simulink model "cordic_mix_v2"  (R2021a)
settings: Solver=VariableStepAuto  StartTime=0.0  StopTime=500  RelTol=1e-3
libraries: xbsIndex_r4 x68, dspsrcs4 x6
settings Model: Creator=user  LastModifiedBy=11037
settings SolverCC: AlgebraicLoopSolver=TrustRegion
settings DataIOCC: ReturnWorkspaceOutputs=off
settings DebuggingCC: SFMachineParentedDataDiag=warning

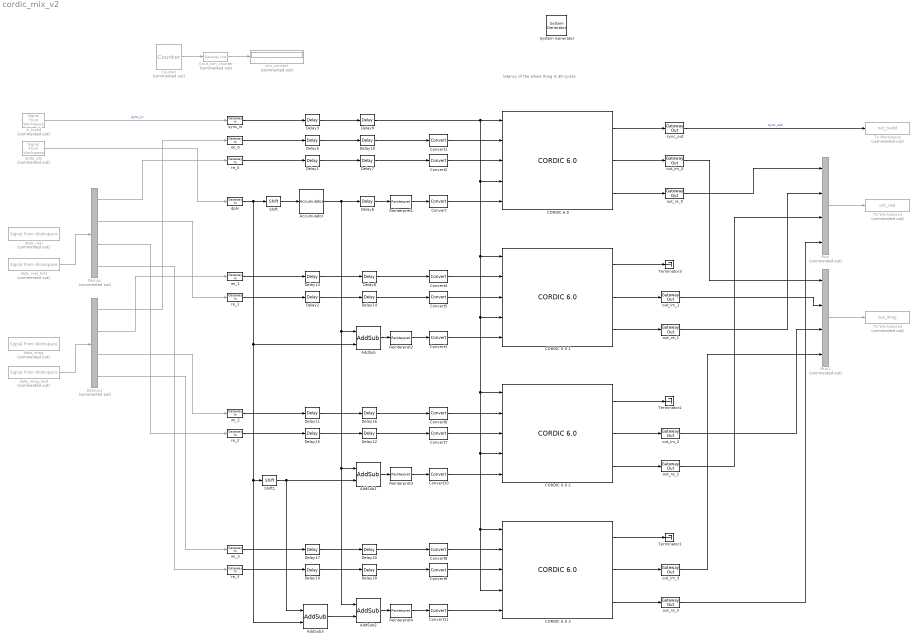
== system cordic_mix_v2 ==
  note: latency of the whole thing is 30 cycles
  " System Generator" : xbsIndex_r4/ System Generator  Tag=genX  xilinxfamily=zynquplusRFSOC  part=xczu28dr  speed=-2-e  package=ffvg1517  synthesis_tool=Vivado  clock_wrapper=Clock Enables  directory=C:/cordic_mix_v2_NL  proj_type=Vivado  Synth_file=Vivado Synthesis Defaults  Impl_file=Vivado Implementation Defaults  testbench=off  simulink_period=1  sysclk_period=10  dcm_input_clock_period=10  incr_netlist=off  trim_vbits=Everywhere in SubSystem  dbl_ovrd=According to Block Masks  core_generation=According to Block Masks  run_coregen=off  deprecated_control=off  eval_field=0  block_type=sysgen
  Accumulator : xbsIndex_r4/Accumulator  operation=Add  n_bits=22  overflow=Wrap  scale=1  rst=off  hasbypass=off  infoeditControl=reset for floating point data type must be asserted for a minimum of 2 cycles  en=off  latency=1  msb_inp=100  msb=100  lsb=-100  use_behavioral_HDL=on  implementation=Fabric  dbl_ovrd=off  block_type=accum
  AddSub : xbsIndex_r4/AddSub  mode=Addition  use_carryin=off  use_carryout=off  en=off  latency=2  precision=User Defined  arith_type=Unsigned  n_bits=22  bin_pt=0  quantization=Truncate  overflow=Wrap  use_behavioral_HDL=off  hw_selection=Fabric  pipelined=off  dbl_ovrd=off  block_type=addsub
  AddSub1 : xbsIndex_r4/AddSub  mode=Addition  use_carryin=off  use_carryout=off  en=off  latency=2  precision=User Defined  arith_type=Unsigned  n_bits=22  bin_pt=0  quantization=Truncate  overflow=Wrap  use_behavioral_HDL=off  hw_selection=Fabric  pipelined=off  dbl_ovrd=off  block_type=addsub
  AddSub2 : xbsIndex_r4/AddSub  mode=Addition  use_carryin=off  use_carryout=off  en=off  latency=2  precision=User Defined  arith_type=Unsigned  n_bits=22  bin_pt=0  quantization=Truncate  overflow=Wrap  use_behavioral_HDL=off  hw_selection=Fabric  pipelined=off  dbl_ovrd=off  block_type=addsub
  AddSub3 : xbsIndex_r4/AddSub  mode=Addition  use_carryin=off  use_carryout=off  en=off  latency=1  precision=User Defined  arith_type=Unsigned  n_bits=22  bin_pt=0  quantization=Truncate  overflow=Wrap  use_behavioral_HDL=off  hw_selection=Fabric  pipelined=off  dbl_ovrd=off  block_type=addsub
  CORDIC 6.0 {,1..3} (4 alike) : xbsIndex_r4/CORDIC 6.0   functional_selection=Rotate  architectural_configuration=Parallel  pipelining_mode=Maximum  data_format=SignedFraction  phase_format=Scaled_Radians  input_width=24  output_width=16  round_mode=Truncate  iterations=18  precision=20  compensation_scaling=LUT_based  coarse_rotation=on  aclken=off  aresetn=off  out_tready=off  cartesian_has_tuser=off  cartesian_has_tlast=off  cartesian_tuser_width=1  phase_has_tuser=off  phase_has_tlast=off  phase_tuser_width=1  out_tlast_behv=Null  flow_control=NonBlocking  optimize_goal=Resources  trim_axipin_name=on  simulation_type=hybrid_sim  simulation_model=sysgen:cordic_v6_0  data_path_portlist={'s_axis_cartesian_tdata_imag', 's_axis_cartesian_tdata_real', 's_axis_phase_tdata_phase', 'm_axis_dout_tdata_imag', 'm_axis_dout_tdata_real', 'm_axis_dout_tdata_phase','m_axis_dout_tdata'}  ip_name=CORDIC  ip_version=6.0  dsptool_ready=true  ipcore_usecache=true  ipcore_useipmodelcache=true  wrapper_available=true  port_translation_map={ 'aclken' => 'en', 'aresetn' => 'rst' }  block_type=cordic_v6_0
      settings: infoedit=CORDIC 6.0
  Convert{,3,10..11} (4 alike) : xbsIndex_r4/Convert  gui_display_data_type=Fixed-point  arith_type="Signed  (2's comp)"  n_bits=24  bin_pt=21  float_type=Single  exp_bits=8  fraction_bits=24  quantization=Truncate  overflow=Flag as error  en=off  latency=0  pipeline=off  dbl_ovrd=off  block_type=convert
  Convert{1..2,4..9} (8 alike) : xbsIndex_r4/Convert  gui_display_data_type=Fixed-point  arith_type="Signed  (2's comp)"  n_bits=24  bin_pt=22  float_type=Single  exp_bits=8  fraction_bits=24  quantization=Truncate  overflow=Flag as error  en=off  latency=0  pipeline=off  dbl_ovrd=off  block_type=convert
  Counter : xbsIndex_r4/Counter  Commented=on  cnt_type=Free Running  cnt_to=Inf  operation=Up  start_count=0  cnt_by_val=1  arith_type=Unsigned  n_bits=24  bin_pt=0  load_pin=off  rst=off  en=off  explicit_period=on  period=1  use_behavioral_HDL=off  implementation=Fabric  dbl_ovrd=off  block_type=counter
  Delay{1..3,5,11,13,15,17,19} (9 alike) : xbsIndex_r4/Delay  rst=off  infoeditControl=Selection of Reset will increase slice count due to use of real FFs and instead of SRLs  en=off  latency=1  reg_retiming=off  dbl_ovrd=off  block_type=delay
  Delay{6..10,12,14,16,18,20} (10 alike) : xbsIndex_r4/Delay  rst=off  infoeditControl=Selection of Reset will increase slice count due to use of real FFs and instead of SRLs  en=off  latency=2  reg_retiming=off  dbl_ovrd=off  block_type=delay
  Demux : Demux  Commented=on
  Demux1 : Demux  Commented=on
  Gout_sim_counter : xbsIndex_r4/Gateway Out  Commented=on  inherit_from_input=on  hdl_port=on  rows=1  columns=1  UseAsDAC=off  DACChannel='1'  interface=None  automatic_assignment=on  address_offset=hex2dec('00')  intf_name=''  intf_description=''  timing_constraint=None  locs_specified=off  LOCs={}  io_standard={}  block_type=gatewayout
  Mux : Mux  Commented=on
  Mux1 : Mux  Commented=on
  Reinterpret{1..4} (4 alike) : xbsIndex_r4/Reinterpret  force_arith_type=on  arith_type="Signed  (2's comp)"  force_bin_pt=on  bin_pt=21  block_type=reinterpret
  Shift : xbsIndex_r4/Shift  shift_dir=Left  shift_bits=2  en=off  latency=0  precision=Full  arith_type="Signed  (2's comp)"  n_bits=16  bin_pt=14  quantization=Truncate  overflow=Wrap  dbl_ovrd=off  block_type=shift
  Shift1 : xbsIndex_r4/Shift  shift_dir=Left  shift_bits=1  en=off  latency=0  precision=Full  arith_type="Signed  (2's comp)"  n_bits=16  bin_pt=14  quantization=Truncate  overflow=Wrap  dbl_ovrd=off  block_type=shift
  Terminator1 : Terminator
  Terminator2 : Terminator
  Terminator3 : Terminator
  To Workspace : ToWorkspace  Commented=on  VariableName=out_tvalid  SampleTime=1
  To Workspace1 : ToWorkspace  Commented=on  VariableName=out_real  SampleTime=1
  To Workspace2 : ToWorkspace  Commented=on  VariableName=out_imag  SampleTime=1
  data_imag : dspsrcs4/Signal From Workspace  Commented=on  X=PSB_out_im_trimmed  Ts=1  nsamps=1  OutputAfterFinalValue=Cyclic repetition  ignoreOrWarnInputAndFrameLengths=off  OutputFrames=off
  data_imag_test : dspsrcs4/Signal From Workspace  Commented=on  X=cordic_test_signal_imag  Ts=1  nsamps=1  OutputAfterFinalValue=Cyclic repetition  ignoreOrWarnInputAndFrameLengths=off  OutputFrames=off
  data_real : dspsrcs4/Signal From Workspace  Commented=on  X=PSB_out_re_trimmed  Ts=1  nsamps=1  OutputAfterFinalValue=Cyclic repetition  ignoreOrWarnInputAndFrameLengths=off  OutputFrames=off
  data_real_test : dspsrcs4/Signal From Workspace  Commented=on  X=cordic_test_signal_real  Ts=1  nsamps=1  OutputAfterFinalValue=Cyclic repetition  ignoreOrWarnInputAndFrameLengths=off  OutputFrames=off
  delta_phi : dspsrcs4/Signal From Workspace  Commented=on  X=dphi  Ts=1  nsamps=1  OutputAfterFinalValue=Holding final value  ignoreOrWarnInputAndFrameLengths=off  OutputFrames=off
  dphi : xbsIndex_r4/Gateway In  gui_display_data_type=Fixed-point  arith_type=Unsigned  n_bits=22  bin_pt=0  preci_type=Single  exp_width=8  frac_width=24  rows=1  columns=1  quantization=Truncate  overflow=Flag as error  period=1  UseAsADC=off  ADCChannel='1'  interface=None  automatic_assignment=on  address_offset=hex2dec('00')  intf_name=''  intf_description=''  default_value=0  timing_constraint=None  locs_specified=off  LOCs={}  io_standard={}  inherit_from_input=off  hdl_port=on  dbl_ovrd=off  block_type=gatewayin
  im_{0..3} (4 alike) : xbsIndex_r4/Gateway In  gui_display_data_type=Fixed-point  arith_type="Signed  (2's comp)"  n_bits=16  bin_pt=15  preci_type=Double  exp_width=8  frac_width=24  rows=1  columns=1  quantization=Truncate  overflow=Flag as error  period=1  UseAsADC=off  ADCChannel='1'  interface=None  automatic_assignment=on  address_offset=hex2dec('00')  intf_name=''  intf_description=''  default_value=0  timing_constraint=None  locs_specified=off  LOCs={}  io_standard={}  inherit_from_input=off  hdl_port=on  dbl_ovrd=off  block_type=gatewayin
  in_tvalid : dspsrcs4/Signal From Workspace  Commented=on  X=1  Ts=1  nsamps=1  OutputAfterFinalValue=Holding final value  ignoreOrWarnInputAndFrameLengths=off  OutputFrames=off
  out_im_{0..3} (4 alike) : xbsIndex_r4/Gateway Out  inherit_from_input=off  hdl_port=on  rows=1  columns=1  UseAsDAC=off  DACChannel='1'  interface=None  automatic_assignment=on  address_offset=hex2dec('00')  intf_name=''  intf_description=''  timing_constraint=None  locs_specified=off  LOCs={}  io_standard={}  block_type=gatewayout
  out_re_{0..3} (4 alike) : xbsIndex_r4/Gateway Out  inherit_from_input=off  hdl_port=on  rows=1  columns=1  UseAsDAC=off  DACChannel='1'  interface=None  automatic_assignment=on  address_offset=hex2dec('00')  intf_name=''  intf_description=''  timing_constraint=None  locs_specified=off  LOCs={}  io_standard={}  block_type=gatewayout
  re_{0..3} (4 alike) : xbsIndex_r4/Gateway In  gui_display_data_type=Fixed-point  arith_type="Signed  (2's comp)"  n_bits=16  bin_pt=15  preci_type=Double  exp_width=8  frac_width=24  rows=1  columns=1  quantization=Truncate  overflow=Flag as error  period=1  UseAsADC=off  ADCChannel='1'  interface=None  automatic_assignment=on  address_offset=hex2dec('00')  intf_name=''  intf_description=''  default_value=0  timing_constraint=None  locs_specified=off  LOCs={}  io_standard={}  inherit_from_input=off  hdl_port=on  dbl_ovrd=off  block_type=gatewayin
  sim_counter : Display  Commented=on
      settings: Format=decimal (Stored Integer)
  sync_in : xbsIndex_r4/Gateway In  gui_display_data_type=Boolean  arith_type=Boolean  n_bits=1  bin_pt=0  preci_type=Single  exp_width=8  frac_width=24  rows=1  columns=1  quantization="Round  (unbiased: +/- Inf)"  overflow=Saturate  period=1  UseAsADC=off  ADCChannel='1'  interface=None  automatic_assignment=on  address_offset=hex2dec('00')  intf_name=''  intf_description=''  default_value=0  timing_constraint=None  locs_specified=off  LOCs={}  io_standard={}  inherit_from_input=off  hdl_port=on  dbl_ovrd=off  block_type=gatewayin
  sync_out : xbsIndex_r4/Gateway Out  inherit_from_input=off  hdl_port=on  rows=1  columns=1  UseAsDAC=off  DACChannel='1'  interface=None  automatic_assignment=on  address_offset=hex2dec('00')  intf_name=''  intf_description=''  timing_constraint=None  locs_specified=off  LOCs={}  io_standard={}  block_type=gatewayout
  wires:
  sync_in/1 -> Delay3/1
  "CORDIC 6.0 "/1 -> sync_out/1
  "CORDIC 6.0 "/2 -> out_im_0/1
  "CORDIC 6.0 "/3 -> out_re_0/1
  out_re_0/1 -> Mux/1
  out_im_0/1 -> Mux1/1
  delta_phi/1 -> dphi/1
  Convert/1 -> "CORDIC 6.0 "/5
  Delay3/1 -> Delay9/1
  Demux/1 -> re_0/1
  Demux1/1 -> im_0/1
  in_tvalid/1 -> sync_in/1  "sync_in"
  sync_out/1 -> To Workspace/1  "sync_out"
  Reinterpret1/1 -> Convert/1
  Delay5/1 -> Delay10/1
  Delay1/1 -> Delay7/1
  im_0/1 -> Delay5/1
  re_0/1 -> Delay1/1
  Convert1/1 -> "CORDIC 6.0 "/2
  Convert2/1 -> "CORDIC 6.0 "/3
  dphi/1 -> Shift/1, AddSub/2, Shift1/1, AddSub3/2
  Delay6/1 -> Reinterpret1/1
  Accumulator/1 -> Delay6/1, AddSub/1, AddSub1/1, AddSub2/1
  Shift/1 -> Accumulator/1
  AddSub/1 -> Reinterpret2/1
  Reinterpret2/1 -> Convert3/1
  Delay7/1 -> Convert2/1
  Delay10/1 -> Convert1/1
  Delay9/1 -> "CORDIC 6.0 "/1, "CORDIC 6.0 "/4, CORDIC 6.0 1/1, CORDIC 6.0 2/4, CORDIC 6.0 3/1, CORDIC 6.0 3/4, CORDIC 6.0 2/1, CORDIC 6.0 1/4
  Delay8/1 -> Convert4/1
  Delay14/1 -> Convert5/1
  Convert5/1 -> CORDIC 6.0 1/3
  Convert4/1 -> CORDIC 6.0 1/2
  re_1/1 -> Delay2/1
  im_1/1 -> Delay13/1
  Delay2/1 -> Delay14/1
  Delay13/1 -> Delay8/1
  Convert3/1 -> CORDIC 6.0 1/5
  Demux1/2 -> im_1/1
  Demux/2 -> re_1/1
  out_im_1/1 -> Mux1/2
  out_re_1/1 -> Mux/2
  CORDIC 6.0 1/2 -> out_im_1/1
  CORDIC 6.0 1/3 -> out_re_1/1
  out_re_2/1 -> Mux/3
  out_im_2/1 -> Mux1/3
  out_re_3/1 -> Mux/4
  out_im_3/1 -> Mux1/4
  CORDIC 6.0 3/2 -> out_im_3/1
  CORDIC 6.0 3/3 -> out_re_3/1
  CORDIC 6.0 3/1 -> Terminator1/1
  CORDIC 6.0 2/3 -> out_re_2/1
  CORDIC 6.0 2/2 -> out_im_2/1
  CORDIC 6.0 2/1 -> Terminator2/1
  CORDIC 6.0 1/1 -> Terminator3/1
  re_2/1 -> Delay15/1
  Delay12/1 -> Convert7/1
  Delay15/1 -> Delay12/1
  Delay11/1 -> Delay16/1
  Convert6/1 -> CORDIC 6.0 2/2
  Demux1/3 -> im_2/1
  Delay16/1 -> Convert6/1
  Convert7/1 -> CORDIC 6.0 2/3
  Demux/3 -> re_2/1
  im_2/1 -> Delay11/1
  re_3/1 -> Delay19/1
  Delay18/1 -> Convert9/1
  Delay19/1 -> Delay18/1
  Delay17/1 -> Delay20/1
  Convert8/1 -> CORDIC 6.0 3/2
  Demux1/4 -> im_3/1
  Delay20/1 -> Convert8/1
  Convert9/1 -> CORDIC 6.0 3/3
  Demux/4 -> re_3/1
  im_3/1 -> Delay17/1
  Reinterpret3/1 -> Convert10/1
  AddSub1/1 -> Reinterpret3/1
  Shift1/1 -> AddSub1/2, AddSub3/1
  AddSub2/1 -> Reinterpret4/1
  Reinterpret4/1 -> Convert11/1
  AddSub3/1 -> AddSub2/2
  Convert11/1 -> CORDIC 6.0 3/5
  Convert10/1 -> CORDIC 6.0 2/5
  Mux/1 -> To Workspace1/1
  Mux1/1 -> To Workspace2/1
  Gout_sim_counter/1 -> sim_counter/1
  Counter/1 -> Gout_sim_counter/1
  data_real_test/1 -> Demux/1
  data_imag_test/1 -> Demux1/1
